simulink model "ifm"  (R2012b)
settings: Solver=ode45  StartTime=0.0  StopTime=.01  RelTol=1e-3
undefined symbols (not defined in the file or in its folder): dfilt, get, Radix
libraries: dsparch4 x2, dspsnks4 x2, commchan3 x1, dspxfrm3 x1, simulink x1
settings Model: Creator=saghafi  LastModifiedBy=Ahmad

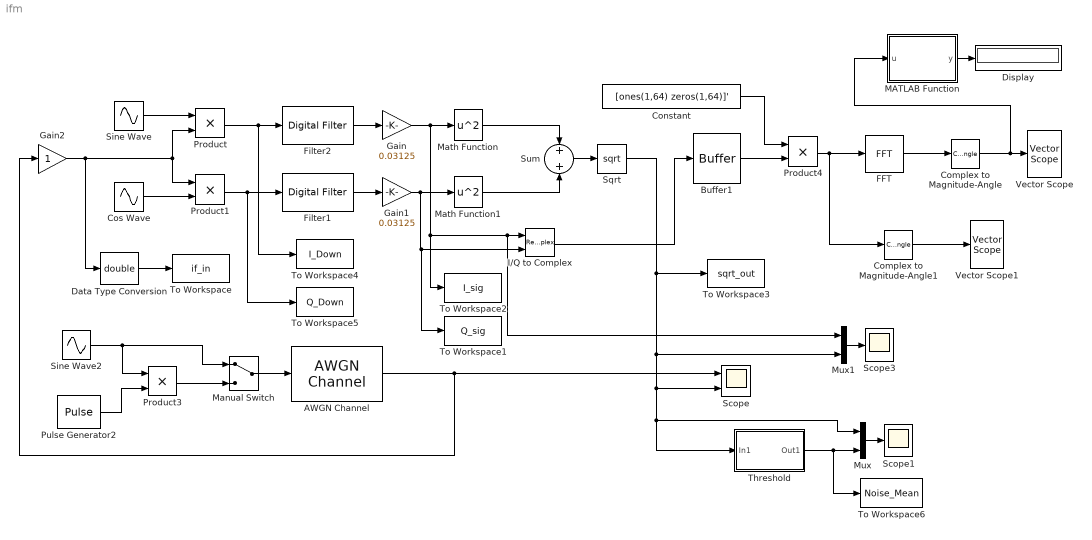
== system ifm ==
  AWGN Channel : commchan3/AWGN Channel  InputProcessing=Inherited (this choice will be removed - see release notes)  seed=67  noiseMode="Signal to noise ratio  (SNR)"  EbNodB=10  EsNodB=10  SNRdB=15  bitsPerSym=1  Ps=0.125  Tsym=1  variance=1
  Buffer1 : Buffer  N=64+64  TreatMby1Signals=One channel
  Complex to Magnitude-Angle : ComplexToMagnitudeAngle  Output=Magnitude
  Complex to Magnitude-Angle1 : ComplexToMagnitudeAngle  Output=Magnitude
  Constant : Constant  Value=[ones(1,64) zeros(1,64)]'  VectorParams1D=off  SampleTime=1/2e6  FramePeriod=1/1e6
      settings: SamplingMode=Frame based
  Cos Wave : Sin  Frequency=2*pi*32e6  Phase=pi/2  SampleTime=1/128e6
  Data Type Conversion : DataTypeConversion  OutDataTypeStr=double
  Display : Display
  FFT : dspxfrm3/FFT  CompMethod=Table lookup  TableOpt=NEW  TableOptActive=Speed  BitRevOrder=off  InheritFFTLength=off  FFTLength=64+64  RowConvenienceOn=on  FFTImplementation=Radix-2  SkipNorm=on  firstCoeffDataTypeStr=Inherit: Same word length as input  firstCoeffLastDataTypeStr=Inherit: Same word length as input  outputMin=[]  outputMax=[]  roundingMode=Floor  overflowMode=off
  Filter1 : dsparch4/Digital Filter  Tag=BlockMethodSubSystem  TypePopup=IIR (poles & zeros)  IIRFiltStruct=Direct form II  AllPoleFiltStruct=Direct form  FIRFiltStruct=Direct form  CoeffSource=Specify via dialog  NumCoeffs=round( [0.028 0.053 0.071 0.053 0.028].*2^20)/2^15  DenCoeffs=round( [1 -2.026 2.148 -1.159 0.279].*2^15)/2^15  BiQuadCoeffs=[1 0.3 0.4 1 0.1 0.2]  LatticeCoeffs=[0.2 0.4]  denIgnore=on  FiltPerSampPopup=One filter per frame  IC=0  ICnum=0  ICden=0  firstCoeffMode=Binary point scaling  firstCoeffWordLength=18  firstCoeffFracLength=15  outputMode=Binary point scaling  outputWordLength=14  outputFracLength=13  accumMode=Binary point scaling  accumWordLength=42  accumFracLength=35  prodOutputMode=Binary point scaling  prodOutputWordLength=42  prodOutputFracLength=35  memoryMode=Binary point scaling  memoryWordLength=24  memoryFracLength=20  roundingMode=Floor  overflowMode=off  ScaleValues=1  scaleValueFracLength=14  stageInFracLength=15  stageOutFracLength=15  FilterSource=Specify via dialog  dfiltObjectName=dfilt.dffir([1 2 1])
  Filter2 : dsparch4/Digital Filter  Tag=BlockMethodSubSystem  TypePopup=IIR (poles & zeros)  IIRFiltStruct=Direct form II  AllPoleFiltStruct=Direct form  FIRFiltStruct=Direct form  CoeffSource=Specify via dialog  NumCoeffs=round( [0.028 0.053 0.071 0.053 0.028].*2^20)/2^15  DenCoeffs=round( [1 -2.026 2.148 -1.159 0.279].*2^15)/2^15  BiQuadCoeffs=[1 0.3 0.4 1 0.1 0.2]  LatticeCoeffs=[0.2 0.4]  denIgnore=on  FiltPerSampPopup=One filter per frame  IC=0  ICnum=0  ICden=0  firstCoeffMode=Binary point scaling  firstCoeffWordLength=18  firstCoeffFracLength=15  outputMode=Binary point scaling  outputWordLength=14  outputFracLength=13  accumMode=Binary point scaling  accumWordLength=42  accumFracLength=35  prodOutputMode=Binary point scaling  prodOutputWordLength=42  prodOutputFracLength=35  memoryMode=Binary point scaling  memoryWordLength=24  memoryFracLength=20  roundingMode=Floor  overflowMode=off  ScaleValues=1  scaleValueFracLength=14  stageInFracLength=15  stageOutFracLength=15  FilterSource=Specify via dialog  dfiltObjectName=dfilt.dffir([1 2 1])
  Gain : Gain  Gain=0.03125
  Gain1 : Gain  Gain=0.03125
  Gain2 : Gain  OutDataTypeStr=fixdt(1,14,13)  RndMeth=Round  SampleTime=1/128e6  SaturateOnIntegerOverflow=on
  I/Q to Complex : RealImagToComplex
  MATLAB Function : MATLAB Function  TreatAsAtomicUnit=on
  Manual Switch : ManualSwitch
  Math Function : Math  Operator=square  SaturateOnIntegerOverflow=on
  Math Function1 : Math  Operator=square  SaturateOnIntegerOverflow=on
  Mux : Mux  Inputs=2
  Mux1 : Mux  Inputs=2
  Product : Product  SaturateOnIntegerOverflow=on  RndMeth=Zero
  Product1 : Product  SaturateOnIntegerOverflow=on  RndMeth=Zero
  Product3 : Product  SampleTime=1/128e6  RndMeth=Zero
  Product4 : Product  RndMeth=Zero
  Pulse Generator2 : DiscretePulseGenerator  PulseType=Time based  Period=20e-6  PulseWidth=4
  Scope : Scope  NumInputPorts=2
      settings: TimeRange=0.02  YMin=0~-5  YMax=8.5~5
  Scope1 : Scope
      settings: TimeRange=0.02  YMin=0  YMax=8.5
  Scope3 : Scope
      settings: TimeRange=0.02  YMin=0  YMax=8.5  SaveName=ScopeData3
  Sine Wave : Sin  Frequency=2*pi*32e6  SampleTime=1/128e6
  Sine Wave2 : Sin  Amplitude=.5  Frequency=2*pi*163.7e6  SampleTime=1/128e6
  Sqrt : Sqrt  SaturateOnIntegerOverflow=on
  Sum : Sum  Inputs=+|+
  Threshold : Subsystem
  To Workspace : ToWorkspace  VariableName=if_in  SampleTime=-1  SaveFormat=Timeseries
  To Workspace1 : ToWorkspace  VariableName=Q_sig  SampleTime=-1  SaveFormat=Timeseries
  To Workspace2 : ToWorkspace  VariableName=I_sig  SampleTime=-1  SaveFormat=Timeseries
  To Workspace3 : ToWorkspace  VariableName=sqrt_out  SampleTime=-1  SaveFormat=Timeseries
  To Workspace4 : ToWorkspace  VariableName=I_Down  SampleTime=-1  SaveFormat=Timeseries
  To Workspace5 : ToWorkspace  VariableName=Q_Down  SampleTime=-1  SaveFormat=Timeseries
  To Workspace6 : ToWorkspace  VariableName=Noise_Mean  SampleTime=-1  SaveFormat=Timeseries
  Vector Scope : dspsnks4/Vector Scope  ScopeProperties=on  Domain=Frequency  HorizSpan=1  DisplayProperties=off  AxisGrid=on  Memory=off  FrameNumber=on  AxisLegend=on  AxisZoom=off  OpenScopeAtSimStart=on  OpenScopeImmediately=off  FigPos=get(0,'defaultfigureposition')  AxisProperties=off  XUnits=Hertz  XRange=[0...Fs]  InheritXIncr=on  XIncr=1  XLabel=Time  XLimit=User-defined  XMin=0  XMax=128000000  XStart=0  YUnits=Magnitude  YLabel=Amplitude  LineProperties=off  LineMarkers=o  LineColors=[0 0 1]  XAxisParamsVer=6.9
      settings: YMin=-50.0064  YMax=-11.244
  Vector Scope1 : dspsnks4/Vector Scope  ScopeProperties=on  Domain=User-defined  HorizSpan=1  DisplayProperties=off  AxisGrid=on  Memory=off  FrameNumber=on  AxisLegend=on  AxisZoom=off  OpenScopeAtSimStart=on  OpenScopeImmediately=off  FigPos=get(0,'defaultfigureposition')  AxisProperties=off  XUnits=Hertz  XRange=[0...Fs]  InheritXIncr=on  XIncr=1  XLabel=Time  XLimit=Auto  XMin=0  XMax=1  XStart=0  YUnits=dB  YLabel=Amplitude  LineProperties=off  LineMarkers=o  XAxisParamsVer=6.9
      settings: YMin=-10  YMax=10
  wires:
  Sine Wave/1 -> Product/1
  Cos Wave/1 -> Product1/2
  Product/1 -> Filter2/1, To Workspace4/1
  Product1/1 -> Filter1/1, To Workspace5/1
  Math Function/1 -> Sum/1
  Math Function1/1 -> Sum/2
  Sum/1 -> Sqrt/1
  FFT/1 -> Complex to Magnitude-Angle/1
  Sqrt/1 -> Mux1/2, Threshold/1(In1), Mux/1, Scope/2, To Workspace3/1
  Pulse Generator2/1 -> Product3/2
  Gain2/1 -> Data Type Conversion/1, Product1/1, Product/2
  Filter2/1 -> Gain/1
  Constant/1 -> Product4/1
  Buffer1/1 -> Product4/2
  Product4/1 -> FFT/1, Complex to Magnitude-Angle1/1
  Complex to Magnitude-Angle1/1 -> Vector Scope1/1
  AWGN Channel/1 -> Gain2/1, Scope/1
  I/Q to Complex/1 -> Buffer1/1
  Sine Wave2/1 -> Manual Switch/1, Product3/1
  Complex to Magnitude-Angle/1 -> MATLAB Function/1(u), Vector Scope/1
  Filter1/1 -> Gain1/1
  Gain/1 -> Mux1/1, I/Q to Complex/1, To Workspace2/1, Math Function/1
  Gain1/1 -> To Workspace1/1, I/Q to Complex/2, Math Function1/1
  Data Type Conversion/1 -> To Workspace/1
  Mux/1 -> Scope1/1
  Threshold/1(Out1) -> To Workspace6/1, Mux/2
  MATLAB Function/1(y) -> Display/1
  Mux1/1 -> Scope3/1
  Product3/1 -> Manual Switch/2
  Manual Switch/1 -> AWGN Channel/1

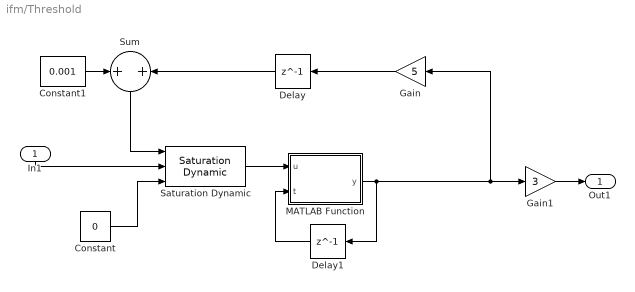
== system ifm/Threshold ==
  In1 : Inport
  Constant : Constant  Value=0  SampleTime=1/128e6
  Constant1 : Constant  Value=0.001  SampleTime=1/128e6
  Delay : Delay  DelayLength=1  InitialCondition=0
  Delay1 : Delay  DelayLength=1  InitialCondition=0
  Gain : Gain  Gain=5
  Gain1 : Gain  Gain=3
  MATLAB Function : MATLAB Function  TreatAsAtomicUnit=on
  Saturation Dynamic : simulink/Discontinuities/Saturation Dynamic  OutMin=[]  OutMax=[]  OutDataTypeStr=Inherit: Same as second input  OutDataType=fixdt(1, 16)  OutScaling=2^-10  DoSatur=off
  Sum : Sum  Inputs=+|+
  Out1 : Outport
  wires:
  Saturation Dynamic/1 -> MATLAB Function/1(u)
  Constant/1 -> Saturation Dynamic/3
  Sum/1 -> Saturation Dynamic/1
  Constant1/1 -> Sum/1
  Delay/1 -> Sum/2
  Gain/1 -> Delay/1
  MATLAB Function/1(y) -> Gain/1, Gain1/1, Delay1/1
  Gain1/1 -> Out1/1
  Delay1/1 -> MATLAB Function/2(t)
  In1/1 -> Saturation Dynamic/2

== matlab function ifm/MATLAB Function ==
  data: u input; y output
function y = fcn(u)

[t i] = max(u);

if i == 1
    i=2;
end;

if i == 128
    i=127;
end;

a = u(i-1);
b = u(i);
c = u(i+1);

p = (a - c) / (2 * (a - 2*b + c));
y = i+p + 160 -1;

== matlab function ifm/Threshold/MATLAB Function ==
  data: u input; y output; t input
function y = fcn(u,t)

    alpha = 2^(-15);
    y = (1 - alpha) * t + alpha * u;
